simulink model "generic_wilmer_och_linnea_medvektorer2016b"  (R2016b)
settings: Solver=ode45  StartTime=0.0  StopTime=inf  RelTol=1e-3  EnableMultiTasking=on
libraries: CarMaker4SL x84, simulink x2
(part 1 of 2)
settings Model: ExtModeAutoUpdateStatusClock=off  Creator=fh  LastModifiedBy=Jeder
settings DataIOCC: LimitDataPoints=on  SaveFormat=Array  SignalLoggingSaveFormat=ModelDataLogs  SignalLoggingName=sigsOut
settings OptimizationCC: BooleanDataType=off  ExpressionDepthLimit=2147483647  InitFltsAndDblsToZero=on  LifeSpan=inf
settings DebuggingCC: SaveWithParameterizedLinksMsg=none  UnderspecifiedInitializationDetection=Classic  MergeDetectMultiDrivingBlocksExec=none  SignalResolutionControl=TryResolveAllWithWarning  MultiTaskDSMMsg=warning  MultiTaskCondExecSysMsg=none  FcnCallInpInsideContextMsg=warning  StateNameClashWarn=warning  SFUnexpectedBacktrackingDiag=warning  SFNoUnconditionalDefaultTransitionDiag=warning  SFExecutionAtInitializationDiag=none
settings HardwareCC: ProdBitPerPointer=32  ProdBitPerSizeT=32  ProdBitPerPtrDiffT=32  ProdLargestAtomicFloat=None  ProdIntDivRoundTo=Undefined  ProdEndianess=Unspecified  ProdWordSize=32  ProdHWDeviceType=32-bit Generic  TargetBitPerPointer=64  TargetBitPerSizeT=64  TargetBitPerPtrDiffT=64  TargetLongLongMode=on  TargetIntDivRoundTo=Zero  TargetEndianess=LittleEndian  TargetWordSize=64  TargetHWDeviceType=MATLAB Host  ProdEqTarget=off
settings ModelReferenceCC: PropagateSignalLabelsOutOfModel=off
settings CodeAppCC: MaxIdLength=63
settings GRTTargetCC: TargetFcnLib=ansi_tfl_tmw.mat  TargetLangStandard=C89/C90 (ANSI)  GeneratePreprocessorConditionals=Disable all  CombineOutputUpdateFcns=off  GRTInterface=on
settings ConfigComp: CovMetricSettings=dw  CovHtmlReporting=on  CovSaveCumulativeToWorkspaceVar=on  CovSaveSingleToWorkspaceVar=on  CovExternalEMLEnable=off

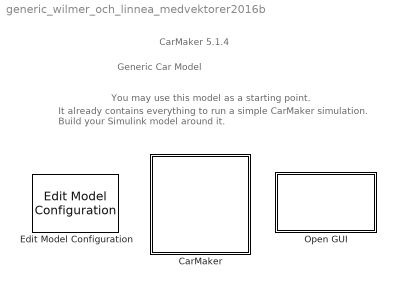
== system generic_wilmer_och_linnea_medvektorer2016b ==
  note: Generic Car Model
  note: You may use this model as a starting point.
  note: It already contains everything to run a simple CarMaker simulation.
      | Build your Simulink model around it.
  note: CarMaker 5.1.4
  CarMaker : Subsystem  TreatAsAtomicUnit=on
      mask Display: image(imread('CarMaker4SLss.bmp'));
  Edit Model Configuration : CarMaker4SL/Edit Model Configuration
  Open GUI : Subsystem  LoadFcn=if ~length(which('cmcmd')), cmenv; end
      settings: OpenFcn=cmblockmagic('gui_fix_display'); CM_Simulink
      mask Display: image(imread('CarMakerGUI.bmp'));

== system generic_wilmer_och_linnea_medvektorer2016b/CarMaker ==
  CM_FIRST : Subsystem
  CM_LAST : Subsystem
  DrivMan : Subsystem
  Ground : Ground
  IPG Vehicle : Subsystem  TreatAsAtomicUnit=on
  Terminator : Terminator
  VehicleControl : Subsystem
  wires:
  DrivMan/2(DrivMan.Out) -> VehicleControl/2(DrivMan.In)
  DrivMan/1(Sync_Out) -> VehicleControl/1(Sync_In)
  CM_FIRST/2(Env.Misc) -> DrivMan/2(Env.Misc)
  CM_FIRST/1(Sync_Out) -> DrivMan/1(Sync_In)
  CM_LAST/1(Sync_Out) -> Terminator/1
  IPG Vehicle/1(Sync_Out) -> CM_LAST/1(Sync_In)
  VehicleControl/1(Sync_Out) -> IPG Vehicle/1(Sync_In)
  VehicleControl/3(VhclCtrl.Steering) -> IPG Vehicle/3(VhclCtrl.Steering)
  VehicleControl/4(Vhcl.Wheel.In) -> IPG Vehicle/4(Vhcl.Wheel.In)
  VehicleControl/5(Vhcl.Misc) -> IPG Vehicle/5(Vhcl.Misc)
  VehicleControl/6(VhclCtrl.Brake) -> IPG Vehicle/6(VhclCtrl.Brake)
  VehicleControl/7(VhclCtrl.PT) -> IPG Vehicle/7(VhclCtrl.PT)
  VehicleControl/2(Vhcl.Model.Source) -> IPG Vehicle/2(Vhcl.Model.Source)
  Ground/1 -> CM_FIRST/1(Sync_In)

== system generic_wilmer_och_linnea_medvektorer2016b/Open GUI ==
  S-Function : S-Function  FunctionName=cm_gui  SFunctionDeploymentMode=off  EnableBusSupport=off

== system generic_wilmer_och_linnea_medvektorer2016b/CarMaker/CM_FIRST ==
  Sync_In : Inport
  Bus Creator1 : BusCreator  Inputs=9
  Demux : Demux  Outputs=9
  Environment : S-Function  FunctionName=CM_Sfun  Parameters='Environment'  SFunctionDeploymentMode=off  EnableBusSupport=off
  IoIn : S-Function  FunctionName=CM_Sfun  Parameters='IoIn'  SFunctionDeploymentMode=off  EnableBusSupport=off
  Sync_Out : Outport
  Env.Misc : Outport  Port=2
  wires:
  Bus Creator1/1 -> Env.Misc/1
  Environment/2 -> Demux/1
  Demux/4 -> Bus Creator1/4  "Env AirHumidity"
  Demux/3 -> Bus Creator1/3  "Env AirPressure"
  Demux/2 -> Bus Creator1/2  "Env AirDensity"
  Demux/1 -> Bus Creator1/1  "Env Temperature"
  Environment/1 -> Sync_Out/1
  IoIn/1 -> Environment/1
  Sync_In/1 -> IoIn/1
  Demux/5 -> Bus Creator1/5  "Env Time"
  Demux/6 -> Bus Creator1/6  "Env SolarRadiation"
  Demux/7 -> Bus Creator1/7  "Env WindVel_tot x"
  Demux/8 -> Bus Creator1/8  "Env WindVel_tot y"
  Demux/9 -> Bus Creator1/9  "Env WindVel_tot z"

== system generic_wilmer_och_linnea_medvektorer2016b/CarMaker/CM_LAST ==
  Sync_In : Inport
  CM_User : S-Function  FunctionName=CM_Sfun  Parameters='CM_User'  SFunctionDeploymentMode=off  EnableBusSupport=off
  IoOut : S-Function  FunctionName=CM_Sfun  Parameters='IoOut'  SFunctionDeploymentMode=off  EnableBusSupport=off
  Sync_Out : Outport
  wires:
  IoOut/1 -> Sync_Out/1
  CM_User/1 -> IoOut/1
  Sync_In/1 -> CM_User/1

== system generic_wilmer_och_linnea_medvektorer2016b/CarMaker/DrivMan ==
  note: There's rarely a reason to override DrivMan signals.
      | Use the VehicleControl interface for this purpose.
  Sync_In : Inport
  Env.Misc : Inport  Port=2
  BusCreator : BusCreator  Inputs=17
  Demux : Demux  Outputs=17
  DrivMan : S-Function  FunctionName=CM_Sfun  Parameters='DrivMan'  SFunctionDeploymentMode=off  EnableBusSupport=off
  Sync_Out : Outport
  DrivMan.Out : Outport  Port=2
  wires:
  Demux/17 -> BusCreator/17  "DrivMan Steering Trq"
  Demux/16 -> BusCreator/16  "DrivMan Steering AngAcc"
  Demux/15 -> BusCreator/15  "DrivMan Steering AngVel"
  Demux/14 -> BusCreator/14  "DrivMan Steering Ang"
  Demux/13 -> BusCreator/13  "DrivMan Gas"
  Demux/12 -> BusCreator/12  "DrivMan Clutch"
  Demux/11 -> BusCreator/11  "DrivMan BrakePark"
  Demux/10 -> BusCreator/10  "DrivMan Brake"
  Demux/9 -> BusCreator/9  "DrivMan GearNo"
  Demux/8 -> BusCreator/8  "DrivMan SelectorCtrl"
  Demux/7 -> BusCreator/7  "DrivMan UserSignal4"
  Demux/6 -> BusCreator/6  "DrivMan UserSignal3"
  Demux/5 -> BusCreator/5  "DrivMan UserSignal2"
  Demux/4 -> BusCreator/4  "DrivMan UserSignal1"
  Demux/3 -> BusCreator/3  "DrivMan UserSignal0"
  Demux/2 -> BusCreator/2  "DrivMan Key"
  Demux/1 -> BusCreator/1  "DrivMan SST"
  Env.Misc/1 -> DrivMan/2
  Sync_In/1 -> DrivMan/1
  DrivMan/1 -> Sync_Out/1
  BusCreator/1 -> DrivMan.Out/1
  DrivMan/2 -> Demux/1

== system generic_wilmer_och_linnea_medvektorer2016b/CarMaker/IPG Vehicle ==
  Sync_In : Inport
  Vhcl.Model.Source : Inport  Port=2
  VhclCtrl.Steering : Inport  Port=3
  Vhcl.Wheel.In : Inport  Port=4
  Vhcl.Misc : Inport  Port=5
  VhclCtrl.Brake : Inport  Port=6
  VhclCtrl.PT : Inport  Port=7
  Brake : Subsystem
  CarAndTrailer : Subsystem
  PowerTrain : Subsystem
  Stop Simulation : Stop
  VehicleSource_BuiltIn : simulink/Logic and Bit Operations/Compare To Constant  relop=~=  const=1  OutDataTypeStr=boolean  ZeroCross=off
  Sync_Out : Outport
  wires:
  VhclCtrl.PT/1 -> PowerTrain/3(VhclCtrl.PT)
  Brake/1(Sync_Out) -> PowerTrain/1(Sync_In)
  CarAndTrailer/1(Sync_Out) -> Brake/1(Sync_In)
  CarAndTrailer/2(Brake.IF.In) -> Brake/2(Brake.IF.In)
  VhclCtrl.Brake/1 -> Brake/3(VhclCtrl.Brake)
  PowerTrain/1(Sync_Out) -> Sync_Out/1
  Vhcl.Misc/1 -> CarAndTrailer/4(Vhcl.Misc)
  Vhcl.Wheel.In/1 -> CarAndTrailer/3(Vhcl.Wheel.In)
  VhclCtrl.Steering/1 -> CarAndTrailer/2(VhclCtrl.Steering)
  Sync_In/1 -> CarAndTrailer/1(Sync_In)
  Vhcl.Model.Source/1 -> VehicleSource_BuiltIn/1
  VehicleSource_BuiltIn/1 -> Stop Simulation/1
  Brake/2(Vhcl.Wheel.PT) -> PowerTrain/2(Vhcl.Wheel.PT)

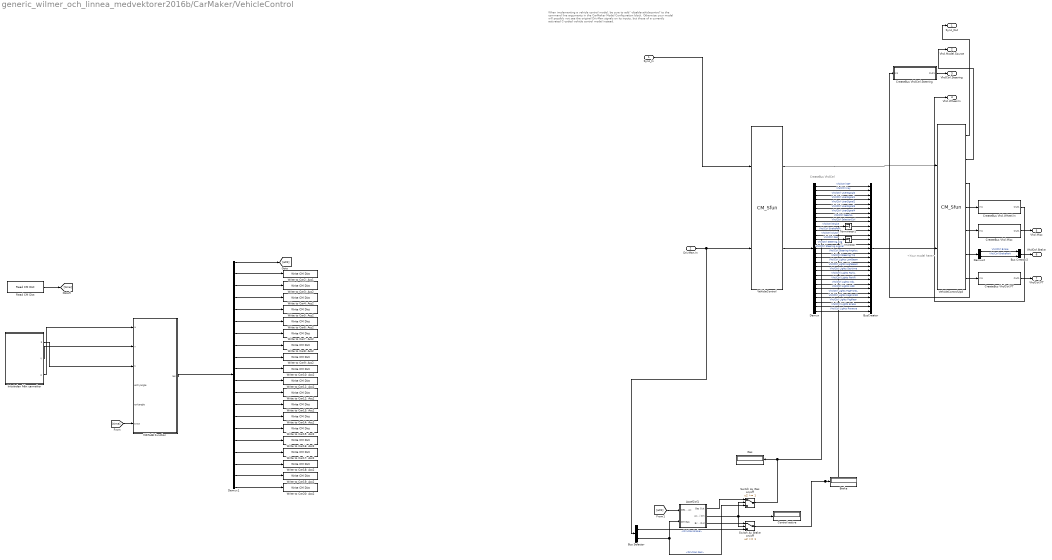
== system generic_wilmer_och_linnea_medvektorer2016b/CarMaker/VehicleControl ==
  note: CreateBus VhclCtrl
  note: <Your model here>
  note: When implementing a vehicle control model,
      | be sure to add '-disablevehiclecontrol' to the command line arguments
      | in the CarMaker Model Configuration block.
      | Otherwise your model will possibly not see the original DrivMan signals
      | on its inputs, but those of a currently activated C-coded vehicle control model instead.
  Sync_In : Inport
  DrivMan.In : Inport  Port=2
  AccelCtrl1 : Subsystem
  Brake : Display
  Bus Creator2 : BusCreator  Inputs=2
  Bus Selector : BusSelector  OutputSignals=DrivMan Brake,DrivMan Gas
  BusCreator : BusCreator  Inputs=29
  Control active : Display
  CreateBus Vhcl.Misc : Subsystem
  CreateBus Vhcl.Wheel.In : Subsystem
  CreateBus VhclCtrl.PT : Subsystem
  CreateBus VhclCtrl.Steering : Subsystem
  Demux : Demux  Outputs=29
  Demux1 : Demux  Outputs=20
  Demux2 : Demux  Outputs=2
  Gas : Display
  Initvärden från carmaker : Subsystem
  MATLAB Function : MATLAB Function  TreatAsAtomicUnit=on
  Read CM Dict : CarMaker4SL/Read CM Dict  xname=Time  xsync=off
  Switch Ax Brake on/off : Switch  Threshold=1  SaturateOnIntegerOverflow=on
  Switch Ax Gas on/off : Switch  Threshold=1  SaturateOnIntegerOverflow=on
  Terminator : Terminator
  Terminator1 : Terminator
  VehicleControl : S-Function  FunctionName=CM_Sfun  Parameters='VehicleControl'  SFunctionDeploymentMode=off  EnableBusSupport=off
  VehicleControlUpd : S-Function  FunctionName=CM_Sfun  Parameters='VehicleControlUpd'  SFunctionDeploymentMode=off  EnableBusSupport=off
  Write to Car10: Acc2 : CarMaker4SL/Write CM Dict  xname=Traffic.T08.LongAcc  xsync=off
  Write to Car11: Acc2 : CarMaker4SL/Write CM Dict  xname=Traffic.T09.LongAcc  xsync=off
  Write to Car12: Acc2 : CarMaker4SL/Write CM Dict  xname=Traffic.T10.LongAcc  xsync=off
  Write to Car13: Acc2 : CarMaker4SL/Write CM Dict  xname=Traffic.T11.LongAcc  xsync=off
  Write to Car14: Acc2 : CarMaker4SL/Write CM Dict  xname=Traffic.T12.LongAcc  xsync=off
  Write to Car15: Acc2 : CarMaker4SL/Write CM Dict  xname=Traffic.T13.LongAcc  xsync=off
  Write to Car16: Acc2 : CarMaker4SL/Write CM Dict  xname=Traffic.T14.LongAcc  xsync=off
  Write to Car17: Acc2 : CarMaker4SL/Write CM Dict  xname=Traffic.T15.LongAcc  xsync=off
  Write to Car18: Acc2 : CarMaker4SL/Write CM Dict  xname=Traffic.T16.LongAcc  xsync=off
  Write to Car19: Acc2 : CarMaker4SL/Write CM Dict  xname=Traffic.T17.LongAcc  xsync=off
  Write to Car20: Acc2 : CarMaker4SL/Write CM Dict  xname=Traffic.T18.LongAcc  xsync=off
  Write to Car2: Acc1 : CarMaker4SL/Write CM Dict  xname=Traffic.T00.LongAcc  xsync=off
  Write to Car3: Acc2 : CarMaker4SL/Write CM Dict  xname=Traffic.T01.LongAcc  xsync=off
  Write to Car4: Acc2 : CarMaker4SL/Write CM Dict  xname=Traffic.T02.LongAcc  xsync=off
  Write to Car5: Acc2 : CarMaker4SL/Write CM Dict  xname=Traffic.T03.LongAcc  xsync=off
  Write to Car6: Acc2 : CarMaker4SL/Write CM Dict  xname=Traffic.T04.LongAcc  xsync=off
  Write to Car7: Acc2 : CarMaker4SL/Write CM Dict  xname=Traffic.T05.LongAcc  xsync=off
  Write to Car8: Acc2 : CarMaker4SL/Write CM Dict  xname=Traffic.T06.LongAcc  xsync=off
  Write to Car9: Acc2 : CarMaker4SL/Write CM Dict  xname=Traffic.T07.LongAcc  xsync=off
  Sync_Out : Outport
  Vhcl.Model.Source : Outport  Port=2
  VhclCtrl.Steering : Outport  Port=3
  Vhcl.Wheel.In : Outport  Port=4
  Vhcl.Misc : Outport  Port=5
  VhclCtrl.Brake : Outport  Port=6
  VhclCtrl.PT : Outport  Port=7
  wires:
  BusCreator/1 -> VehicleControlUpd/2
  VehicleControlUpd/2 -> Vhcl.Model.Source/1
  VehicleControlUpd/4 -> CreateBus Vhcl.Wheel.In/1(In1)
  VehicleControlUpd/5 -> CreateBus Vhcl.Misc/1(In1)
  VehicleControlUpd/6 -> Demux2/1
  VehicleControlUpd/7 -> CreateBus VhclCtrl.PT/1(In1)
  VehicleControlUpd/3 -> CreateBus VhclCtrl.Steering/1(In1)
  CreateBus Vhcl.Misc/1(Out1) -> Vhcl.Misc/1
  CreateBus Vhcl.Wheel.In/1(Out1) -> Vhcl.Wheel.In/1
  VehicleControl/1 -> VehicleControlUpd/1
  Sync_In/1 -> VehicleControl/1
  CreateBus VhclCtrl.PT/1(Out1) -> VhclCtrl.PT/1
  Bus Creator2/1 -> VhclCtrl.Brake/1
  CreateBus VhclCtrl.Steering/1(Out1) -> VhclCtrl.Steering/1
  VehicleControlUpd/1 -> Sync_Out/1
  Demux2/2 -> Bus Creator2/2  "VhclCtrl BrakePark"
  Demux2/1 -> Bus Creator2/1  "VhclCtrl Brake"
  Demux/29 -> BusCreator/29  "VhclCtrl Lights Reverse"
  Demux/28 -> BusCreator/28  "VhclCtrl Lights Brake"
  Demux/27 -> BusCreator/27  "VhclCtrl Lights FogRear"
  Demux/26 -> BusCreator/26  "VhclCtrl Lights FogFrontR"
  Demux/25 -> BusCreator/25  "VhclCtrl Lights FogFrontL"
  Demux/24 -> BusCreator/24  "VhclCtrl Lights IndR"
  Demux/23 -> BusCreator/23  "VhclCtrl Lights IndL"
  Demux/22 -> BusCreator/22  "VhclCtrl Lights ParkR"
  Demux/21 -> BusCreator/21  "VhclCtrl Lights ParkL"
  Demux/20 -> BusCreator/20  "VhclCtrl Lights Daytime"
  Demux/19 -> BusCreator/19  "VhclCtrl Lights HighBeam"
  Demux/18 -> BusCreator/18  "VhclCtrl Lights LowBeam"
  Demux/17 -> BusCreator/17  "VhclCtrl Steering Trq"
  Demux/16 -> BusCreator/16  "VhclCtrl Steering AngAcc"
  Demux/15 -> BusCreator/15  "VhclCtrl Steering AngVel"
  Demux/14 -> BusCreator/14  "VhclCtrl Steering Ang"
  Demux/13 -> Terminator/1  "VhclCtrl Gas"
  Demux/12 -> BusCreator/12  "VhclCtrl Clutch"
  Demux/11 -> BusCreator/11  "VhclCtrl BrakePark"
  Demux/10 -> Terminator1/1  "VhclCtrl Brake"
  Demux/9 -> BusCreator/9  "VhclCtrl SelectorCtrl"
  Demux/8 -> BusCreator/8  "VhclCtrl GearNo"
  Demux/7 -> BusCreator/7  "VhclCtrl UserSignal4"
  Demux/6 -> BusCreator/6  "VhclCtrl UserSignal3"
  Demux/5 -> BusCreator/5  "VhclCtrl UserSignal2"
  Demux/4 -> BusCreator/4  "VhclCtrl UserSignal1"
  Demux/3 -> BusCreator/3  "VhclCtrl UserSignal0"
  Demux/2 -> BusCreator/2  "VhclCtrl Key"
  Demux/1 -> BusCreator/1  "VhclCtrl SST"
  VehicleControl/2 -> Demux/1
  DrivMan.In/1 -> VehicleControl/2, Bus Selector/1
  AccelCtrl1/2(AxCtrl On) -> Switch Ax Gas on/off/2, Control active/1, Switch Ax Brake on/off/2
  Bus Selector/1 -> Switch Ax Brake on/off/3  "<DrivMan Brake>"
  AccelCtrl1/3(Brake Out) -> Switch Ax Brake on/off/1
  AccelCtrl1/1(Gas Out) -> Switch Ax Gas on/off/1
  Bus Selector/2 -> Switch Ax Gas on/off/3, AccelCtrl1/2(DM Gas)  "<DrivMan Gas>"
  [a01] -> AccelCtrl1/1(Desired Ax)
  Switch Ax Gas on/off/1 -> BusCreator/13, Gas/1
  Switch Ax Brake on/off/1 -> Brake/1, BusCreator/10
  MATLAB Function/1(res) -> Demux1/1
  Initvärden från carmaker/1("S ") -> MATLAB Function/3(s)
  Initvärden från carmaker/2("V ") -> MATLAB Function/2(v)
  Initvärden från carmaker/3("A ") -> MATLAB Function/1(a)
  Demux1/1 -> [a01]
  Demux1/2 -> Write to Car2: Acc1/1
  Demux1/3 -> Write to Car3: Acc2/1
  Demux1/4 -> Write to Car4: Acc2/1
  Demux1/5 -> Write to Car5: Acc2/1
  Demux1/6 -> Write to Car6: Acc2/1
  Demux1/7 -> Write to Car7: Acc2/1
  Demux1/8 -> Write to Car8: Acc2/1
  Demux1/9 -> Write to Car9: Acc2/1
  Demux1/10 -> Write to Car10: Acc2/1
  Demux1/11 -> Write to Car11: Acc2/1
  Demux1/12 -> Write to Car12: Acc2/1
  Demux1/13 -> Write to Car13: Acc2/1
  Demux1/14 -> Write to Car14: Acc2/1
  Demux1/15 -> Write to Car15: Acc2/1
  Demux1/16 -> Write to Car16: Acc2/1
  Demux1/17 -> Write to Car17: Acc2/1
  Demux1/18 -> Write to Car18: Acc2/1
  Demux1/19 -> Write to Car19: Acc2/1
  Demux1/20 -> Write to Car20: Acc2/1
  Read CM Dict/1 -> [time]
  [time] -> MATLAB Function/6(time)

== system generic_wilmer_och_linnea_medvektorer2016b/CarMaker/IPG Vehicle/Brake ==
  note: <Your model here>
  note: When replacing the entire braking system,
      | be sure to add '-disablebrake' to the command line arguments
      | in the CarMaker Model Configuration block.
  Sync_In : Inport
  Brake.IF.In : Inport  Port=2
  VhclCtrl.Brake : Inport  Port=3
  Brake : S-Function  FunctionName=CM_Sfun  Parameters='Brake'  SFunctionDeploymentMode=off  EnableBusSupport=off
  BrakeUpd : S-Function  FunctionName=CM_Sfun  Parameters='BrakeUpd'  SFunctionDeploymentMode=off  EnableBusSupport=off
  BusCreator : BusCreator  Inputs=12
  CreateBus Vhcl.Wheel.PT : Subsystem
  Demux : Demux  Outputs=12
  Sync_Out : Outport
  Vhcl.Wheel.PT : Outport  Port=2
  wires:
  BrakeUpd/1 -> Sync_Out/1
  Brake/1 -> BrakeUpd/1  "Sync"
  Brake.IF.In/1 -> Brake/2
  VhclCtrl.Brake/1 -> Brake/3
  Brake/2 -> Demux/1
  BusCreator/1 -> BrakeUpd/2
  Sync_In/1 -> Brake/1
  Demux/12 -> BusCreator/12  "Brake IF Trq_Reg_trg RR"
  Demux/11 -> BusCreator/11  "Brake IF Trq_Reg_trg RL"
  Demux/10 -> BusCreator/10  "Brake IF Trq_Reg_trg FR"
  Demux/9 -> BusCreator/9  "Brake IF Trq_Reg_trg FL"
  Demux/8 -> BusCreator/8  "Brake IF Trq_PB RR"
  Demux/7 -> BusCreator/7  "Brake IF Trq_PB RL"
  Demux/6 -> BusCreator/6  "Brake IF Trq_PB FR"
  Demux/5 -> BusCreator/5  "Brake IF Trq_PB FL"
  Demux/4 -> BusCreator/4  "Brake IF Trq_WB RR"
  Demux/3 -> BusCreator/3  "Brake IF Trq_WB RL"
  Demux/2 -> BusCreator/2  "Brake IF Trq_WB FR"
  Demux/1 -> BusCreator/1  "Brake IF Trq_WB FL"
  BrakeUpd/2 -> CreateBus Vhcl.Wheel.PT/1(In)
  CreateBus Vhcl.Wheel.PT/1(Out) -> Vhcl.Wheel.PT/1

== system generic_wilmer_och_linnea_medvektorer2016b/CarMaker/IPG Vehicle/CarAndTrailer ==
  Sync_In : Inport
  VhclCtrl.Steering : Inport  Port=2
  Vhcl.Wheel.In : Inport  Port=3
  Vhcl.Misc : Inport  Port=4
  CarAndTrailerUpd : Subsystem
  Forces : Subsystem
  Ground : Ground
  Kinematics : Subsystem
  Kinetics : Subsystem
  Steering : Subsystem
  Terminator : Terminator
  Terminator1 : Terminator
  Trailer : Subsystem
  Sync_Out : Outport
  Brake.IF.In : Outport  Port=2
  wires:
  Trailer/9(Car.Hitch.FrcTrq) -> CarAndTrailerUpd/9(Car.Hitch.FrcTrq)
  Trailer/8(Vhcl.Wheel.RR) -> CarAndTrailerUpd/8(Vhcl.Wheel.RR)
  Trailer/7(Vhcl.Wheel.RL) -> CarAndTrailerUpd/7(Vhcl.Wheel.RL)
  Trailer/6(Vhcl.Wheel.FR) -> CarAndTrailerUpd/6(Vhcl.Wheel.FR)
  Trailer/5(Vhcl.Wheel.FL) -> CarAndTrailerUpd/5(Vhcl.Wheel.FL)
  Trailer/4(Vhcl.PoI) -> CarAndTrailerUpd/4(Vhcl.PoI)
  Trailer/3(Vhcl.Motion) -> CarAndTrailerUpd/3(Vhcl.Motion)
  Trailer/2(Vhcl.Steering) -> CarAndTrailerUpd/2(Vhcl.Steering)
  Trailer/1(Sync_Out) -> CarAndTrailerUpd/1(Sync_In)
  CarAndTrailerUpd/2(Brake.IF.In) -> Brake.IF.In/1
  CarAndTrailerUpd/1(Sync_Out) -> Sync_Out/1
  Vhcl.Misc/1 -> Terminator1/1
  Vhcl.Wheel.In/1 -> Terminator/1
  Kinetics/6(WheelCarrier.Misc) -> Trailer/6(WheelCarrier.Misc)
  Kinetics/5(Car.Trq_T2W) -> Trailer/5(Car.Trq_T2W)
  Steering/2(Steer.IF) -> Kinematics/2(Steer.IF)
  Kinetics/4(Car.Fr1) -> Trailer/4(Car.Fr1)
  Kinetics/3(Car.Hitch) -> Trailer/3(Car.Hitch)
  Kinetics/2(Trailer.Load) -> Trailer/2(Trailer.Load)
  VhclCtrl.Steering/1 -> Steering/2(VhclCtrl.Steering)
  Sync_In/1 -> Steering/1(Sync_In)
  Steering/1(Sync_Out) -> Kinematics/1(Sync_In)
  Kinetics/1(Sync_Out) -> Trailer/1(Sync_In)
  Ground/1 -> CarAndTrailerUpd/10(Vhcl.Fr1A)
  Forces/11(FStabi) -> Kinetics/11(FStabi)
  Forces/10(FDamp) -> Kinetics/10(FDamp)
  Forces/9(FSpring) -> Kinetics/9(FSpring)
  Forces/8(TireRR_Out) -> Kinetics/8(TireRR.Out)
  Forces/7(TireRL_Out) -> Kinetics/7(TireRL.Out)
  Forces/6(TireFR_Out) -> Kinetics/6(TireFR.Out)
  Forces/5(TireFL_Out) -> Kinetics/5(TireFL.Out)
  Forces/4(Car.Load) -> Kinetics/4(Car.Load)
  Forces/2(Car.Virtual) -> Kinetics/2(Car.Virtual)
  Kinematics/6(lSpring) -> Forces/6(lSpring)
  Kinematics/7(vDamp) -> Forces/7(vDamp)
  Forces/3(Car.Aero) -> Kinetics/3(Car.Aero)
  Forces/1(Sync_Out) -> Kinetics/1(Sync_In)
  Kinematics/5(TireRR_In) -> Forces/5(TireRR_In)
  Kinematics/4(TireRL_In) -> Forces/4(TireRL_In)
  Kinematics/3(TireFR_In) -> Forces/3(TireFR_In)
  Kinematics/2(TireFL_In) -> Forces/2(TireFL_In)
  Kinematics/1(Sync_Out) -> Forces/1(Sync_In)
  Kinematics/8(lStabi) -> Forces/8(lStabi)
  Forces/12(FBuf) -> Kinetics/12(FBuf)
  Kinematics/9(lBuf) -> Forces/9(lBuf)

== system generic_wilmer_och_linnea_medvektorer2016b/CarMaker/IPG Vehicle/PowerTrain ==
  note: When replacing the entire powertrain,
      | be sure to add '-disablepowertrain' to the command line arguments
      | in the CarMaker Model Configuration block.
  note: <Your model here>
  Sync_In : Inport
  Vhcl.Wheel.PT : Inport  Port=2
  VhclCtrl.PT : Inport  Port=3
  BusCreator : BusCreator  Inputs=40
  Demux : Demux  Outputs=40
  PowerTrain : S-Function  FunctionName=CM_Sfun  Parameters='PowerTrain'  SFunctionDeploymentMode=off  EnableBusSupport=off
  PowerTrainUpd : S-Function  FunctionName=CM_Sfun  Parameters='PowerTrainUpd'  SFunctionDeploymentMode=off  EnableBusSupport=off
  Sync_Out : Outport
  wires:
  Sync_In/1 -> PowerTrain/1
  PowerTrain/2 -> Demux/1
  PowerTrainUpd/1 -> Sync_Out/1
  PowerTrain/1 -> PowerTrainUpd/1  "Sync"
  BusCreator/1 -> PowerTrainUpd/2
  Demux/1 -> BusCreator/1  "PT IF Ignition"
  Demux/2 -> BusCreator/2  "PT IF OperationState"
  Demux/3 -> BusCreator/3  "PT IF OperationError"
  Demux/4 -> BusCreator/4  "PT IF GearNo"
  Demux/5 -> BusCreator/5  "PT IF Engine_rotv"
  Demux/6 -> BusCreator/6  "PT IF Engine_Trq (EngineControl)"
  Demux/7 -> BusCreator/7  "PT IF Trq_Supp2Bdy1 x"
  Demux/8 -> BusCreator/8  "PT IF Trq_Supp2Bdy1 y"
  Demux/9 -> BusCreator/9  "PT IF Trq_Supp2Bdy1 z"
  Demux/10 -> BusCreator/10  "PT IF Trq_Supp2BdyEng x"
  Demux/11 -> BusCreator/11  "PT IF Trq_Supp2BdyEng y"
  Demux/12 -> BusCreator/12  "PT IF DL_iDiff_mean"
  Demux/13 -> BusCreator/13  "PT IF WFL rot"
  Demux/14 -> BusCreator/14  "PT IF WFL rotv"
  Demux/15 -> BusCreator/15  "PT IF WFL Trq_B2W"
  Demux/16 -> BusCreator/16  "PT IF WFL Trq_Drive"
  Demux/17 -> BusCreator/17  "PT IF WFL Trq_Supp2WC"
  Demux/18 -> BusCreator/18  "PT IF WFL Trq_BrakeReg"
  Demux/19 -> BusCreator/19  "PT IF WFL Trq_BrakeReg_max"
  Demux/20 -> BusCreator/20  "PT IF WFR rot"
  Demux/21 -> BusCreator/21  "PT IF WFR rotv"
  Demux/22 -> BusCreator/22  "PT IF WFR Trq_B2W"
  Demux/23 -> BusCreator/23  "PT IF WFR Trq_Drive"
  Demux/24 -> BusCreator/24  "PT IF WFR Trq_Supp2WC"
  Demux/25 -> BusCreator/25  "PT IF WFR Trq_BrakeReg"
  Demux/26 -> BusCreator/26  "PT IF WFR Trq_BrakeReg_max"
  Demux/27 -> BusCreator/27  "PT IF WRL rot"
  Demux/28 -> BusCreator/28  "PT IF WRL rotv"
  Demux/29 -> BusCreator/29  "PT IF WRL Trq_B2W"
  Demux/30 -> BusCreator/30  "PT IF WRL Trq_Drive"
  Demux/31 -> BusCreator/31  "PT IF WRL Trq_Supp2WC"
  Demux/32 -> BusCreator/32  "PT IF WRL Trq_BrakeReg"
  Demux/33 -> BusCreator/33  "PT IF WRL Trq_BrakeReg_max"
  Demux/34 -> BusCreator/34  "PT IF WRR rot"
  Demux/35 -> BusCreator/35  "PT IF WRR rotv"
  Demux/36 -> BusCreator/36  "PT IF WRR Trq_B2W"
  Demux/37 -> BusCreator/37  "PT IF WRR Trq_Drive"
  Demux/38 -> BusCreator/38  "PT IF WRR Trq_Supp2WC"
  Demux/39 -> BusCreator/39  "PT IF WRR Trq_BrakeReg"
  Demux/40 -> BusCreator/40  "PT IF WRR Trq_BrakeReg_max"
  VhclCtrl.PT/1 -> PowerTrain/3
  Vhcl.Wheel.PT/1 -> PowerTrain/2

== system generic_wilmer_och_linnea_medvektorer2016b/CarMaker/VehicleControl/AccelCtrl1 ==
  note: x
  note: x
  Desired Ax : Inport
  DM Gas : Inport  Port=2
  Brake if -1<x<0 : Saturate  UpperLimit=0  LowerLimit=-1
  Compare To Constant : simulink/Logic and Bit Operations/Compare To Constant  relop=~=  const=0  OutDataTypeStr=boolean
  Gain : Gain  Gain=-1  SaturateOnIntegerOverflow=on  OutDataTypeStr=Inherit: Same as input  ParamDataTypeStr=Inherit: Same as input
  Gas  if 0<=x<=1 : Saturate  UpperLimit=1  LowerLimit=0
  PI-Controller : Subsystem
  "controlled process variable " : Subsystem
  Gas Out : Outport
  AxCtrl On : Outport  Port=2
  Brake Out : Outport  Port=3
  wires:
  Compare To Constant/1 -> AxCtrl On/1, PI-Controller/3(AxCtrl On)
  Brake if -1<x<0/1 -> Gain/1
  Gas  if 0<=x<=1/1 -> Gas Out/1
  PI-Controller/1(Gas or Brake) -> Gas  if 0<=x<=1/1, Brake if -1<x<0/1
  DM Gas/1 -> PI-Controller/2(DM_Gas)
  "controlled process variable "/1(delta ax) -> PI-Controller/1(delta_ax)
  Gain/1 -> Brake Out/1
  Desired Ax/1 -> "controlled process variable "/1(desired ax), Compare To Constant/1

== system generic_wilmer_och_linnea_medvektorer2016b/CarMaker/VehicleControl/CreateBus Vhcl.Misc ==
  In1 : Inport
  Bus Creator5 : BusCreator  Inputs=11
  Demux5 : Demux  Outputs=11
  Out1 : Outport
  wires:
  Demux5/11 -> Bus Creator5/11  "Vhcl Wind_vel_0 z"
  Demux5/10 -> Bus Creator5/10  "Vhcl Wind_vel_0 y"
  Demux5/9 -> Bus Creator5/9  "Vhcl Wind_vel_0 x"
  Demux5/8 -> Bus Creator5/8  "Vhcl DL2BdyEng y"
  Demux5/7 -> Bus Creator5/7  "Vhcl DL2BdyEng x"
  Demux5/6 -> Bus Creator5/6  "Vhcl TrqDL2Bdy1B z"
  Demux5/5 -> Bus Creator5/5  "Vhcl TrqDL2Bdy1B y"
  Demux5/4 -> Bus Creator5/4  "Vhcl TrqDL2Bdy1B x"
  Demux5/3 -> Bus Creator5/3  "Vhcl Trq_DL2Bdy1 z"
  In1/1 -> Demux5/1
  Bus Creator5/1 -> Out1/1
  Demux5/2 -> Bus Creator5/2  "Vhcl Trq_DL2Bdy1 y"
  Demux5/1 -> Bus Creator5/1  "Vhcl Trq_DL2Bdy1 x"

== system generic_wilmer_och_linnea_medvektorer2016b/CarMaker/VehicleControl/CreateBus Vhcl.Wheel.In ==
  In1 : Inport
  Bus Creator1 : BusCreator  Inputs=12
  Demux1 : Demux  Outputs=12
  Out1 : Outport
  wires:
  Demux1/12 -> Bus Creator1/12  "Vhcl Wheel RR rotv"
  Demux1/11 -> Bus Creator1/11  "Vhcl Wheel RR Trq_DL2WC"
  Demux1/10 -> Bus Creator1/10  "Vhcl Wheel RR Trq_B2WC"
  Demux1/9 -> Bus Creator1/9  "Vhcl Wheel RL rotv"
  Demux1/8 -> Bus Creator1/8  "Vhcl Wheel RL Trq_DL2WC"
  Demux1/7 -> Bus Creator1/7  "Vhcl Wheel RL Trq_B2WC"
  Demux1/6 -> Bus Creator1/6  "Vhcl Wheel FR rotv"
  Demux1/5 -> Bus Creator1/5  "Vhcl Wheel FR Trq_DL2WC"
  Demux1/4 -> Bus Creator1/4  "Vhcl Wheel FR Trq_B2WC"
  Demux1/3 -> Bus Creator1/3  "Vhcl Wheel FL rotv"
  In1/1 -> Demux1/1
  Bus Creator1/1 -> Out1/1
  Demux1/2 -> Bus Creator1/2  "Vhcl Wheel FL Trq_DL2WC"
  Demux1/1 -> Bus Creator1/1  "Vhcl Wheel FL Trq_B2WC"

== system generic_wilmer_och_linnea_medvektorer2016b/CarMaker/VehicleControl/CreateBus VhclCtrl.PT ==
  In1 : Inport
  BusCreator : BusCreator  Inputs=11
  Demux : Demux  Outputs=11
  Out1 : Outport
  wires:
  In1/1 -> Demux/1
  BusCreator/1 -> Out1/1
  Demux/1 -> BusCreator/1  "VhclCtrl SST"
  Demux/2 -> BusCreator/2  "VhclCtrl Key"
  Demux/3 -> BusCreator/3  "VhclCtrl UserSignal0"
  Demux/4 -> BusCreator/4  "VhclCtrl UserSignal1"
  Demux/5 -> BusCreator/5  "VhclCtrl UserSignal2"
  Demux/6 -> BusCreator/6  "VhclCtrl UserSignal3"
  Demux/7 -> BusCreator/7  "VhclCtrl UserSignal4"
  Demux/8 -> BusCreator/8  "VhclCtrl GearNo"
  Demux/9 -> BusCreator/9  "VhclCtrl SelectorCtrl"
  Demux/10 -> BusCreator/10  "VhclCtrl Clutch"
  Demux/11 -> BusCreator/11  "VhclCtrl Gas"

== system generic_wilmer_och_linnea_medvektorer2016b/CarMaker/VehicleControl/CreateBus VhclCtrl.Steering ==
  In1 : Inport
  Bus Creator : BusCreator  Inputs=5
  Demux : Demux  Outputs=5
  Out1 : Outport
  wires:
  In1/1 -> Demux/1
  Bus Creator/1 -> Out1/1
  Demux/1 -> Bus Creator/1  "VhclCtrl Steering Ang"
  Demux/5 -> Bus Creator/5  "VhclCtrl Steering ByTrq"
  Demux/3 -> Bus Creator/3  "VhclCtrl Steering AngAcc"
  Demux/2 -> Bus Creator/2  "VhclCtrl Steering AngVel"
  Demux/4 -> Bus Creator/4  "VhclCtrl Steering Trq"

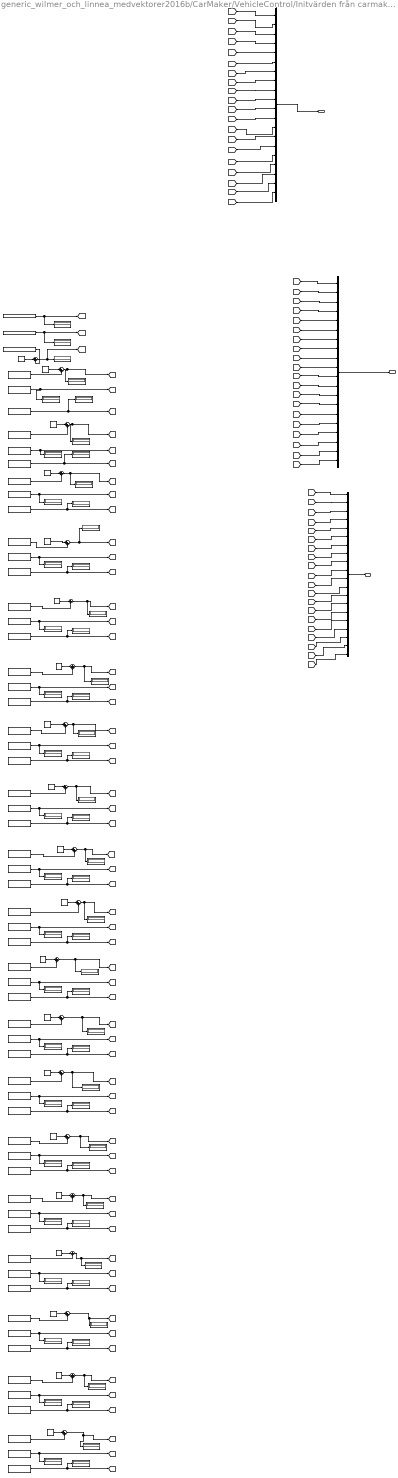
== system generic_wilmer_och_linnea_medvektorer2016b/CarMaker/VehicleControl/Initvärden från carmaker ==
  Constant{,1..19} (20 alike) : Constant  Value=-145
  Display{,1..56} (57 alike) : Display
  Mux : Mux  Inputs=20
  Mux1 : Mux  Inputs=20
  Mux2 : Mux  Inputs=20
  Read CM acceleration : CarMaker4SL/Read CM Dict  xname=Car.ax  xsync=off
  "Read CM position " : CarMaker4SL/Read CM Dict  xname=Car.Road.sRoad  xsync=off
  Read CM velocity : CarMaker4SL/Read CM Dict  xname=Car.vx  xsync=off
  Read Car10 acc : CarMaker4SL/Read CM Dict  xname=Traffic.T08.LongAcc  xsync=off
  Read Car10 dist : CarMaker4SL/Read CM Dict  xname=Traffic.T08.sRoad  xsync=off
  Read Car10 vel : CarMaker4SL/Read CM Dict  xname=Traffic.T08.LongVel  xsync=off
  Read Car11 acc : CarMaker4SL/Read CM Dict  xname=Traffic.T09.LongAcc  xsync=off
  Read Car11 dist : CarMaker4SL/Read CM Dict  xname=Traffic.T09.sRoad  xsync=off
  Read Car11 vel : CarMaker4SL/Read CM Dict  xname=Traffic.T09.LongVel  xsync=off
  Read Car12 acc : CarMaker4SL/Read CM Dict  xname=Traffic.T10.LongAcc  xsync=off
  Read Car12 dist : CarMaker4SL/Read CM Dict  xname=Traffic.T10.sRoad  xsync=off
  Read Car12 vel : CarMaker4SL/Read CM Dict  xname=Traffic.T10.LongVel  xsync=off
  Read Car13 acc : CarMaker4SL/Read CM Dict  xname=Traffic.T11.LongAcc  xsync=off
  Read Car13 dist : CarMaker4SL/Read CM Dict  xname=Traffic.T11.sRoad  xsync=off
  Read Car13 vel : CarMaker4SL/Read CM Dict  xname=Traffic.T11.LongVel  xsync=off
  Read Car14 acc : CarMaker4SL/Read CM Dict  xname=Traffic.T12.LongAcc  xsync=off
  Read Car14 dist : CarMaker4SL/Read CM Dict  xname=Traffic.T12.sRoad  xsync=off
  Read Car14 vel : CarMaker4SL/Read CM Dict  xname=Traffic.T12.LongVel  xsync=off
  Read Car15 acc : CarMaker4SL/Read CM Dict  xname=Traffic.T13.LongAcc  xsync=off
  Read Car15 dist : CarMaker4SL/Read CM Dict  xname=Traffic.T13.sRoad  xsync=off
  Read Car15 vel : CarMaker4SL/Read CM Dict  xname=Traffic.T13.LongVel  xsync=off
  Read Car16 acc : CarMaker4SL/Read CM Dict  xname=Traffic.T14.LongAcc  xsync=off
  Read Car16 dist : CarMaker4SL/Read CM Dict  xname=Traffic.T14.sRoad  xsync=off
  Read Car16 vel : CarMaker4SL/Read CM Dict  xname=Traffic.T14.LongVel  xsync=off
  Read Car17 acc : CarMaker4SL/Read CM Dict  xname=Traffic.T15.LongAcc  xsync=off
  Read Car17 dist : CarMaker4SL/Read CM Dict  xname=Traffic.T15.sRoad  xsync=off
  Read Car17 vel : CarMaker4SL/Read CM Dict  xname=Traffic.T15.LongVel  xsync=off
  Read Car18 acc : CarMaker4SL/Read CM Dict  xname=Traffic.T16.LongAcc  xsync=off
  Read Car18 dist : CarMaker4SL/Read CM Dict  xname=Traffic.T16.sRoad  xsync=off
  Read Car18 vel : CarMaker4SL/Read CM Dict  xname=Traffic.T16.LongVel  xsync=off
  Read Car19 acc : CarMaker4SL/Read CM Dict  xname=Traffic.T17.LongAcc  xsync=off
  Read Car19 dist : CarMaker4SL/Read CM Dict  xname=Traffic.T17.sRoad  xsync=off
  Read Car19 vel : CarMaker4SL/Read CM Dict  xname=Traffic.T17.LongVel  xsync=off
  Read Car2 acc : CarMaker4SL/Read CM Dict  xname=Traffic.T00.LongAcc  xsync=off
  Read Car2 dist : CarMaker4SL/Read CM Dict  xname=Traffic.T00.sRoad  xsync=off
  Read Car2 m/s : CarMaker4SL/Read CM Dict  xname=Traffic.T00.LongVel  xsync=off
  Read Car20 acc : CarMaker4SL/Read CM Dict  xname=Traffic.T18.LongAcc  xsync=off
  Read Car20 dist : CarMaker4SL/Read CM Dict  xname=Traffic.T18.sRoad  xsync=off
  Read Car20 vel : CarMaker4SL/Read CM Dict  xname=Traffic.T18.LongVel  xsync=off
  Read Car3 acc : CarMaker4SL/Read CM Dict  xname=Traffic.T01.LongAcc  xsync=off
  Read Car3 dist : CarMaker4SL/Read CM Dict  xname=Traffic.T01.sRoad  xsync=off
  Read Car3 vel : CarMaker4SL/Read CM Dict  xname=Traffic.T01.LongVel  xsync=off
  Read Car4 acc : CarMaker4SL/Read CM Dict  xname=Traffic.T02.LongAcc  xsync=off
  Read Car4 dist : CarMaker4SL/Read CM Dict  xname=Traffic.T02.sRoad  xsync=off
  Read Car4 vel : CarMaker4SL/Read CM Dict  xname=Traffic.T02.LongVel  xsync=off
  Read Car5 acc5 : CarMaker4SL/Read CM Dict  xname=Traffic.T03.LongAcc  xsync=off
  Read Car5 dist : CarMaker4SL/Read CM Dict  xname=Traffic.T03.sRoad  xsync=off
  Read Car5 vel5 : CarMaker4SL/Read CM Dict  xname=Traffic.T03.LongVel  xsync=off
  Read Car6 acc : CarMaker4SL/Read CM Dict  xname=Traffic.T04.LongAcc  xsync=off
  Read Car6 dist : CarMaker4SL/Read CM Dict  xname=Traffic.T04.sRoad  xsync=off
  Read Car6 vel : CarMaker4SL/Read CM Dict  xname=Traffic.T04.LongVel  xsync=off
  Read Car7 acc1 : CarMaker4SL/Read CM Dict  xname=Traffic.T05.LongAcc  xsync=off
  Read Car7 dist1 : CarMaker4SL/Read CM Dict  xname=Traffic.T05.sRoad  xsync=off
  Read Car7 vel1 : CarMaker4SL/Read CM Dict  xname=Traffic.T05.LongVel  xsync=off
  Read Car8 acc : CarMaker4SL/Read CM Dict  xname=Traffic.T06.LongAcc  xsync=off
  Read Car8 dist : CarMaker4SL/Read CM Dict  xname=Traffic.T06.sRoad  xsync=off
  Read Car8 vel : CarMaker4SL/Read CM Dict  xname=Traffic.T06.LongVel  xsync=off
  Read Car9 acc : CarMaker4SL/Read CM Dict  xname=Traffic.T07.LongAcc  xsync=off
  Read Car9 dist : CarMaker4SL/Read CM Dict  xname=Traffic.T07.sRoad  xsync=off
  Read Car9 vel : CarMaker4SL/Read CM Dict  xname=Traffic.T07.LongVel  xsync=off
  Sum{,1..19} (20 alike) : Sum  Inputs=|++
  pos : Display
  vx1 : Display
  vx2 : Display
  "S " : Outport
  "V " : Outport  Port=2
  "A " : Outport  Port=3
  wires:
  Read Car2 acc/1 -> [a2], Display/1
  Read Car4 vel/1 -> [v4], Display6/1
  Read Car4 acc/1 -> [a4], Display7/1
  Read Car3 acc/1 -> [a3], Display5/1
  Read Car3 vel/1 -> Display4/1, [v3]
  Read Car2 m/s/1 -> Display2/1, [v2]
  Read Car2 dist/1 -> Sum1/2
  Read Car3 dist/1 -> Sum2/2
  Read Car4 dist/1 -> Sum3/2
  Read Car5 vel5/1 -> [v5], Display9/1
  Read Car5 acc5/1 -> [a5], Display10/1
  Read Car5 dist/1 -> Sum4/2
  Read Car6 vel/1 -> [v6], Display12/1
  Read Car6 acc/1 -> [a6], Display13/1
  Read Car7 vel1/1 -> [v7], Display15/1
  Read Car7 acc1/1 -> [a7], Display16/1
  Read Car8 vel/1 -> [v8], Display18/1
  Read Car8 acc/1 -> [a8], Display19/1
  Read Car8 dist/1 -> Sum7/2
  Read Car9 vel/1 -> [v9], Display21/1
  Read Car9 acc/1 -> [a9], Display22/1
  Read Car10 vel/1 -> [v10], Display24/1
  Read Car10 acc/1 -> [a10], Display25/1
  Read Car10 dist/1 -> Sum9/2
  Read Car11 vel/1 -> [v11], Display27/1
  Read Car11 acc/1 -> [a11], Display28/1
  Read Car11 dist/1 -> Sum10/2
  Read Car12 vel/1 -> [v12], Display30/1
  Read Car12 acc/1 -> [a12], Display31/1
  Read Car12 dist/1 -> Sum11/2
  Read Car13 vel/1 -> [v13], Display33/1
  Read Car13 acc/1 -> [a13], Display34/1
  Read Car13 dist/1 -> Sum12/2
  Read Car14 vel/1 -> [v14], Display36/1
  Read Car14 acc/1 -> [a14], Display37/1
  Read Car14 dist/1 -> Sum13/2
  Read Car15 vel/1 -> [v15], Display39/1
  Read Car15 acc/1 -> [a15], Display40/1
  Read Car15 dist/1 -> Sum14/2
  Read Car16 vel/1 -> [v16], Display42/1
  Read Car16 acc/1 -> [a16], Display43/1
  Read Car16 dist/1 -> Sum15/2
  Read Car17 vel/1 -> [v17], Display45/1
  Read Car17 acc/1 -> [a17], Display46/1
  Read Car17 dist/1 -> Sum16/2
  Read Car18 vel/1 -> [v18], Display48/1
  Read Car18 acc/1 -> [a18], Display49/1
  Read Car18 dist/1 -> Sum17/2
  Read Car19 vel/1 -> [v19], Display51/1
  Read Car19 acc/1 -> [a19], Display52/1
  Read Car19 dist/1 -> Sum18/2
  Read Car20 vel/1 -> [v20], Display54/1
  Read Car20 acc/1 -> [a20], Display55/1
  Read Car20 dist/1 -> Sum19/2
  Mux/1 -> "S "/1
  Mux1/1 -> "V "/1
  [s2] -> Mux/2
  [s3] -> Mux/3
  [s8] -> Mux/8
  [s18] -> Mux/18
  [s6] -> Mux/6
  [s19] -> Mux/19
  [s13] -> Mux/13
  [s7] -> Mux/7
  [s4] -> Mux/4
  [s17] -> Mux/17
  [s12] -> Mux/12
  [s11] -> Mux/11
  [s20] -> Mux/20
  [s10] -> Mux/10
  [s16] -> Mux/16
  [s5] -> Mux/5
  [s14] -> Mux/14
  [s15] -> Mux/15
  [s9] -> Mux/9
  [v15] -> Mux1/15
  [v5] -> Mux1/5
  [v20] -> Mux1/20
  [v12] -> Mux1/12
  [v7] -> Mux1/7
  [v2] -> Mux1/2
  [v9] -> Mux1/9
  [v18] -> Mux1/18
  [v17] -> Mux1/17
  [v16] -> Mux1/16
  [v10] -> Mux1/10
  [v3] -> Mux1/3
  [v11] -> Mux1/11
  [v1] -> Mux1/1
  [v8] -> Mux1/8
  [v13] -> Mux1/13
  [v14] -> Mux1/14
  [v4] -> Mux1/4
  [v19] -> Mux1/19
  [v6] -> Mux1/6
  [a2] -> Mux2/2
  [a3] -> Mux2/3
  [a4] -> Mux2/4
  [a5] -> Mux2/5
  [a6] -> Mux2/6
  [a7] -> Mux2/7
  [a8] -> Mux2/8
  [a9] -> Mux2/9
  [a10] -> Mux2/10
  [a11] -> Mux2/11
  [a12] -> Mux2/12
  [a13] -> Mux2/13
  [a14] -> Mux2/14
  [a15] -> Mux2/15
  [a16] -> Mux2/16
  [a17] -> Mux2/17
  [a18] -> Mux2/18
  [a19] -> Mux2/19
  [a20] -> Mux2/20
  Mux2/1 -> "A "/1
  Read CM acceleration/1 -> [a1], vx1/1
  Read CM velocity/1 -> [v1], vx2/1
  [s1] -> Mux/1
  [a1] -> Mux2/1
  Constant/1 -> Sum/1
  "Read CM position "/1 -> Sum/2
  Sum/1 -> pos/1, [s1]
  Constant1/1 -> Sum1/1
  Sum1/1 -> Display1/1, [s2]
  Constant2/1 -> Sum2/1
  Sum2/1 -> Display3/1, [s3]
  Constant3/1 -> Sum3/1
  Sum3/1 -> Display8/1, [s4]
  Constant4/1 -> Sum4/1
  Sum4/1 -> Display11/1, [s5]
  Constant5/1 -> Sum5/1
  Sum5/1 -> Display14/1, [s6]
  Read Car6 dist/1 -> Sum5/2
  Constant6/1 -> Sum6/1
  Read Car7 dist1/1 -> Sum6/2
  Sum6/1 -> Display17/1, [s7]
  Constant7/1 -> Sum7/1
  Sum7/1 -> Display20/1, [s8]
  Constant8/1 -> Sum8/1
  Read Car9 dist/1 -> Sum8/2
  Sum8/1 -> Display23/1, [s9]
  Constant9/1 -> Sum9/1
  Sum9/1 -> Display26/1, [s10]
  Constant10/1 -> Sum10/1
  Sum10/1 -> Display29/1, [s11]
  Constant11/1 -> Sum11/1
  Sum11/1 -> Display32/1, [s12]
  Constant12/1 -> Sum12/1
  Sum12/1 -> Display35/1, [s13]
  Constant13/1 -> Sum13/1
  Sum13/1 -> Display38/1, [s14]
  Constant14/1 -> Sum14/1
  Sum14/1 -> Display41/1, [s15]
  Constant15/1 -> Sum15/1
  Sum15/1 -> Display44/1, [s16]
  Constant16/1 -> Sum16/1
  Sum16/1 -> Display47/1, [s17]
  Constant17/1 -> Sum17/1
  Sum17/1 -> Display50/1, [s18]
  Constant18/1 -> Sum18/1
  Sum18/1 -> Display53/1, [s19]
  Constant19/1 -> Sum19/1
  Sum19/1 -> Display56/1, [s20]

== system generic_wilmer_och_linnea_medvektorer2016b/CarMaker/IPG Vehicle/Brake/CreateBus Vhcl.Wheel.PT ==
  In : Inport
  BusCreator : BusCreator  Inputs=16
  Demux : Demux  Outputs=16
  Out : Outport
  wires:
  Demux/16 -> BusCreator/16  "Vhcl Wheel RR WhlBearing"
  Demux/15 -> BusCreator/15  "Vhcl Wheel RR Trq_T2W"
  Demux/14 -> BusCreator/14  "Vhcl Wheel RR Trq_BrakeReg_trg"
  Demux/13 -> BusCreator/13  "Vhcl Wheel RR Trq_Brake"
  Demux/12 -> BusCreator/12  "Vhcl Wheel RL WhlBearing"
  Demux/11 -> BusCreator/11  "Vhcl Wheel RL Trq_T2W"
  Demux/10 -> BusCreator/10  "Vhcl Wheel RL Trq_BrakeReg_trg"
  Demux/9 -> BusCreator/9  "Vhcl Wheel RL Trq_Brake"
  Demux/8 -> BusCreator/8  "Vhcl Wheel FR WhlBearing"
  Demux/7 -> BusCreator/7  "Vhcl Wheel FR Trq_T2W"
  Demux/6 -> BusCreator/6  "Vhcl Wheel FR Trq_BrakeReg_trg"
  Demux/5 -> BusCreator/5  "Vhcl Wheel FR Trq_Brake"
  Demux/4 -> BusCreator/4  "Vhcl Wheel FL WhlBearing"
  Demux/3 -> BusCreator/3  "Vhcl Wheel FL Trq_T2W"
  Demux/2 -> BusCreator/2  "Vhcl Wheel FL Trq_BrakeReg_trg"
  Demux/1 -> BusCreator/1  "Vhcl Wheel FL Trq_Brake"
  BusCreator/1 -> Out/1
  In/1 -> Demux/1

== system generic_wilmer_och_linnea_medvektorer2016b/CarMaker/IPG Vehicle/CarAndTrailer/CarAndTrailerUpd ==
  Sync_In : Inport
  Vhcl.Steering : Inport  Port=2
  Vhcl.Motion : Inport  Port=3
  Vhcl.PoI : Inport  Port=4
  Vhcl.Wheel.FL : Inport  Port=5
  Vhcl.Wheel.FR : Inport  Port=6
  Vhcl.Wheel.RL : Inport  Port=7
  Vhcl.Wheel.RR : Inport  Port=8
  Car.Hitch.FrcTrq : Inport  Port=9
  Vhcl.Fr1A : Inport  Port=10
  CarAndTrailerUpd : S-Function  FunctionName=CM_Sfun  Parameters='CarAndTrUpd'  SFunctionDeploymentMode=off  EnableBusSupport=off
  CreateBus Brake.IF.In : Subsystem
  Sync_Out : Outport
  Brake.IF.In : Outport  Port=2
  wires:
  Vhcl.Fr1A/1 -> CarAndTrailerUpd/10  "user vehicle only"
  Vhcl.Steering/1 -> CarAndTrailerUpd/2
  Vhcl.Motion/1 -> CarAndTrailerUpd/3
  Vhcl.PoI/1 -> CarAndTrailerUpd/4
  Vhcl.Wheel.FL/1 -> CarAndTrailerUpd/5
  Vhcl.Wheel.FR/1 -> CarAndTrailerUpd/6
  Car.Hitch.FrcTrq/1 -> CarAndTrailerUpd/9
  Vhcl.Wheel.RR/1 -> CarAndTrailerUpd/8
  Vhcl.Wheel.RL/1 -> CarAndTrailerUpd/7
  CarAndTrailerUpd/2 -> CreateBus Brake.IF.In/1(In)
  CreateBus Brake.IF.In/1(Out) -> Brake.IF.In/1
  CarAndTrailerUpd/1 -> Sync_Out/1
  Sync_In/1 -> CarAndTrailerUpd/1

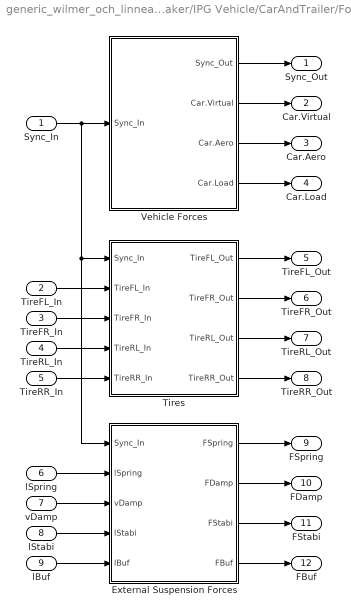
== system generic_wilmer_och_linnea_medvektorer2016b/CarMaker/IPG Vehicle/CarAndTrailer/Forces ==
  Sync_In : Inport
  TireFL_In : Inport  Port=2
  TireFR_In : Inport  Port=3
  TireRL_In : Inport  Port=4
  TireRR_In : Inport  Port=5
  lSpring : Inport  Port=6
  vDamp : Inport  Port=7
  lStabi : Inport  Port=8
  lBuf : Inport  Port=9
  External Suspension Forces : Subsystem
  Tires : Subsystem
  Vehicle Forces : Subsystem
  Sync_Out : Outport
  Car.Virtual : Outport  Port=2
  Car.Aero : Outport  Port=3
  Car.Load : Outport  Port=4
  TireFL_Out : Outport  Port=5
  TireFR_Out : Outport  Port=6
  TireRL_Out : Outport  Port=7
  TireRR_Out : Outport  Port=8
  FSpring : Outport  Port=9
  FDamp : Outport  Port=10
  FStabi : Outport  Port=11
  FBuf : Outport  Port=12
  wires:
  External Suspension Forces/4(FBuf) -> FBuf/1
  lBuf/1 -> External Suspension Forces/5(lBuf)
  Tires/4(TireRR_Out) -> TireRR_Out/1
  Tires/3(TireRL_Out) -> TireRL_Out/1
  Tires/2(TireFR_Out) -> TireFR_Out/1
  Tires/1(TireFL_Out) -> TireFL_Out/1
  TireRR_In/1 -> Tires/5(TireRR_In)
  TireRL_In/1 -> Tires/4(TireRL_In)
  TireFR_In/1 -> Tires/3(TireFR_In)
  Sync_In/1 -> External Suspension Forces/1(Sync_In), Tires/1(Sync_In), Vehicle Forces/1(Sync_In)
  Vehicle Forces/1(Sync_Out) -> Sync_Out/1
  TireFL_In/1 -> Tires/2(TireFL_In)
  Vehicle Forces/2(Car.Virtual) -> Car.Virtual/1
  Vehicle Forces/3(Car.Aero) -> Car.Aero/1
  Vehicle Forces/4(Car.Load) -> Car.Load/1
  lSpring/1 -> External Suspension Forces/2(lSpring)
  External Suspension Forces/2(FDamp) -> FDamp/1
  vDamp/1 -> External Suspension Forces/3(vDamp)
  lStabi/1 -> External Suspension Forces/4(lStabi)
  External Suspension Forces/3(FStabi) -> FStabi/1
  External Suspension Forces/1(FSpring) -> FSpring/1

== system generic_wilmer_och_linnea_medvektorer2016b/CarMaker/IPG Vehicle/CarAndTrailer/Kinematics ==
  Sync_In : Inport
  Steer.IF : Inport  Port=2
  Kinematics : S-Function  FunctionName=CM_Sfun  Parameters='Kinematics'  SFunctionDeploymentMode=off  EnableBusSupport=off
  Sync_Out : Outport
  TireFL_In : Outport  Port=2
  TireFR_In : Outport  Port=3
  TireRL_In : Outport  Port=4
  TireRR_In : Outport  Port=5
  lSpring : Outport  Port=6
  vDamp : Outport  Port=7
  lStabi : Outport  Port=8
  lBuf : Outport  Port=9
  wires:
  Kinematics/9 -> lBuf/1
  Kinematics/8 -> lStabi/1
  Kinematics/2 -> TireFL_In/1
  Kinematics/3 -> TireFR_In/1
  Kinematics/4 -> TireRL_In/1
  Kinematics/5 -> TireRR_In/1
  Kinematics/6 -> lSpring/1
  Kinematics/7 -> vDamp/1
  Sync_In/1 -> Kinematics/1
  Kinematics/1 -> Sync_Out/1
  Steer.IF/1 -> Kinematics/2

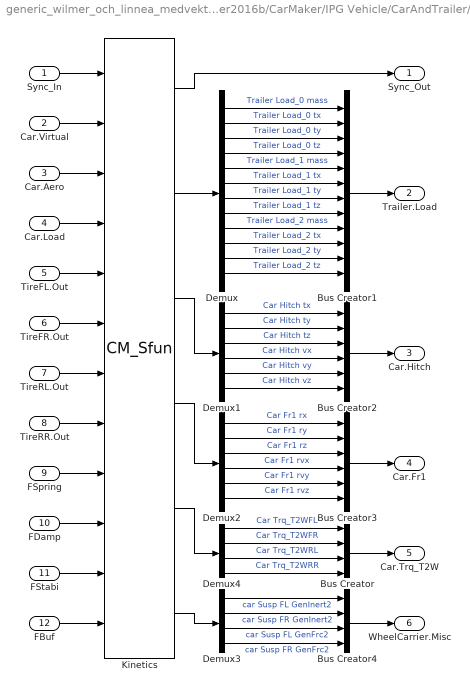
== system generic_wilmer_och_linnea_medvektorer2016b/CarMaker/IPG Vehicle/CarAndTrailer/Kinetics ==
  Sync_In : Inport
  Car.Virtual : Inport  Port=2
  Car.Aero : Inport  Port=3
  Car.Load : Inport  Port=4
  TireFL.Out : Inport  Port=5
  TireFR.Out : Inport  Port=6
  TireRL.Out : Inport  Port=7
  TireRR.Out : Inport  Port=8
  FSpring : Inport  Port=9
  FDamp : Inport  Port=10
  FStabi : Inport  Port=11
  FBuf : Inport  Port=12
  Bus Creator : BusCreator  Inputs=4
  Bus Creator1 : BusCreator  Inputs=12
  Bus Creator2 : BusCreator  Inputs=6
  Bus Creator3 : BusCreator  Inputs=6
  Bus Creator4 : BusCreator  Inputs=4
  Demux : Demux  Outputs=12
  Demux1 : Demux  Outputs=6
  Demux2 : Demux  Outputs=6
  Demux3 : Demux
  Demux4 : Demux
  Kinetics : S-Function  FunctionName=CM_Sfun  Parameters='Kinetics'  SFunctionDeploymentMode=off  EnableBusSupport=off
  Sync_Out : Outport
  Trailer.Load : Outport  Port=2
  Car.Hitch : Outport  Port=3
  Car.Fr1 : Outport  Port=4
  Car.Trq_T2W : Outport  Port=5
  WheelCarrier.Misc : Outport  Port=6
  wires:
  FBuf/1 -> Kinetics/12
  Sync_In/1 -> Kinetics/1
  Kinetics/1 -> Sync_Out/1
  Car.Aero/1 -> Kinetics/3
  Car.Virtual/1 -> Kinetics/2
  Bus Creator1/1 -> Trailer.Load/1
  Demux/1 -> Bus Creator1/1  "Trailer Load_0 mass"
  Demux/2 -> Bus Creator1/2  "Trailer Load_0 tx"
  Demux/3 -> Bus Creator1/3  "Trailer Load_0 ty"
  Demux/4 -> Bus Creator1/4  "Trailer Load_0 tz"
  Kinetics/2 -> Demux/1
  Demux/5 -> Bus Creator1/5  "Trailer Load_1 mass"
  Demux/6 -> Bus Creator1/6  "Trailer Load_1 tx"
  Demux/7 -> Bus Creator1/7  "Trailer Load_1 ty"
  Demux/8 -> Bus Creator1/8  "Trailer Load_1 tz"
  Demux/9 -> Bus Creator1/9  "Trailer Load_2 mass"
  Demux/10 -> Bus Creator1/10  "Trailer Load_2 tx"
  Demux/11 -> Bus Creator1/11  "Trailer Load_2 ty"
  Demux/12 -> Bus Creator1/12  "Trailer Load_2 tz"
  Demux1/1 -> Bus Creator2/1  "Car Hitch tx"
  Demux1/2 -> Bus Creator2/2  "Car Hitch ty"
  Demux1/3 -> Bus Creator2/3  "Car Hitch tz"
  Demux1/4 -> Bus Creator2/4  "Car Hitch vx"
  Demux1/5 -> Bus Creator2/5  "Car Hitch vy"
  Demux1/6 -> Bus Creator2/6  "Car Hitch vz"
  Kinetics/3 -> Demux1/1
  Bus Creator2/1 -> Car.Hitch/1
  Demux2/1 -> Bus Creator3/1  "Car Fr1 rx"
  Demux2/2 -> Bus Creator3/2  "Car Fr1 ry"
  Demux2/3 -> Bus Creator3/3  "Car Fr1 rz"
  Demux2/4 -> Bus Creator3/4  "Car Fr1 rvx"
  Demux2/5 -> Bus Creator3/5  "Car Fr1 rvy"
  Demux2/6 -> Bus Creator3/6  "Car Fr1 rvz"
  Bus Creator3/1 -> Car.Fr1/1
  Kinetics/4 -> Demux2/1
  Car.Load/1 -> Kinetics/4
  Demux3/1 -> Bus Creator4/1  "car Susp FL GenInert2"
  Demux3/2 -> Bus Creator4/2  "car Susp FR GenInert2"
  Demux3/3 -> Bus Creator4/3  "car Susp FL GenFrc2"
  Demux3/4 -> Bus Creator4/4  "car Susp FR GenFrc2"
  Bus Creator4/1 -> WheelCarrier.Misc/1
  Bus Creator/1 -> Car.Trq_T2W/1
  Demux4/4 -> Bus Creator/4  "Car Trq_T2WRR"
  Demux4/3 -> Bus Creator/3  "Car Trq_T2WRL"
  Demux4/2 -> Bus Creator/2  "Car Trq_T2WFR"
  Demux4/1 -> Bus Creator/1  "Car Trq_T2WFL"
  TireFL.Out/1 -> Kinetics/5
  TireFR.Out/1 -> Kinetics/6
  TireRL.Out/1 -> Kinetics/7
  TireRR.Out/1 -> Kinetics/8
  FSpring/1 -> Kinetics/9
  FDamp/1 -> Kinetics/10
  FStabi/1 -> Kinetics/11
  Kinetics/6 -> Demux3/1
  Kinetics/5 -> Demux4/1

== system generic_wilmer_och_linnea_medvektorer2016b/CarMaker/IPG Vehicle/CarAndTrailer/Steering ==
  note: When replacing the entire steering system,
      | be sure to add '-disablesteering' to the command line arguments
      | in the CarMaker Model Configuration block.
  Sync_In : Inport
  VhclCtrl.Steering : Inport  Port=2
  Bus Creator1 : BusCreator  Inputs=16
  Bus Creator2 : BusCreator  Inputs=4
  Demux : Demux  Outputs=20
  Steering : S-Function  FunctionName=CM_Sfun  Parameters='Steering'  SFunctionDeploymentMode=off  EnableBusSupport=off
  Terminator : Terminator
  Sync_Out : Outport
  Steer.IF : Outport  Port=2
  wires:
  Bus Creator1/1 -> Steer.IF/1
  Steering/2 -> Demux/1
  Demux/8 -> Bus Creator1/8  "Steering IF AssistTrqPin"
  Demux/7 -> Bus Creator1/7  "Steering IF AssistTrqCol"
  Demux/6 -> Bus Creator1/6  "Steering IF AssistFrc"
  Demux/20 -> Bus Creator2/4  "Steering IF R Inert"
  Demux/17 -> Bus Creator2/1  "Steering IF L Frc"
  Demux/18 -> Bus Creator2/2  "Steering IF L Inert"
  Demux/19 -> Bus Creator2/3  "Steering IF R Frc"
  Bus Creator2/1 -> Terminator/1  "Steer IF (in)"
  Demux/16 -> Bus Creator1/16  "Steering IF R iSteer2q"
  Demux/9 -> Bus Creator1/9  "Steering IF L q"
  Demux/10 -> Bus Creator1/10  "Steering IF L qp"
  Demux/11 -> Bus Creator1/11  "Steering IF L qpp"
  Demux/12 -> Bus Creator1/12  "Steering IF L iSteer2q"
  Demux/13 -> Bus Creator1/13  "Steering IF R q"
  Demux/14 -> Bus Creator1/14  "Steering IF R qp"
  Demux/15 -> Bus Creator1/15  "Steering IF R qpp"
  VhclCtrl.Steering/1 -> Steering/2
  Steering/1 -> Sync_Out/1
  Sync_In/1 -> Steering/1
  Demux/1 -> Bus Creator1/1  "Steering IF Ang"
  Demux/2 -> Bus Creator1/2  "Steering IF AngVel"
  Demux/3 -> Bus Creator1/3  "Steering IF AngAcc"
  Demux/4 -> Bus Creator1/4  "Steering IF Trq"
  Demux/5 -> Bus Creator1/5  "Steering IF TrqStatic"

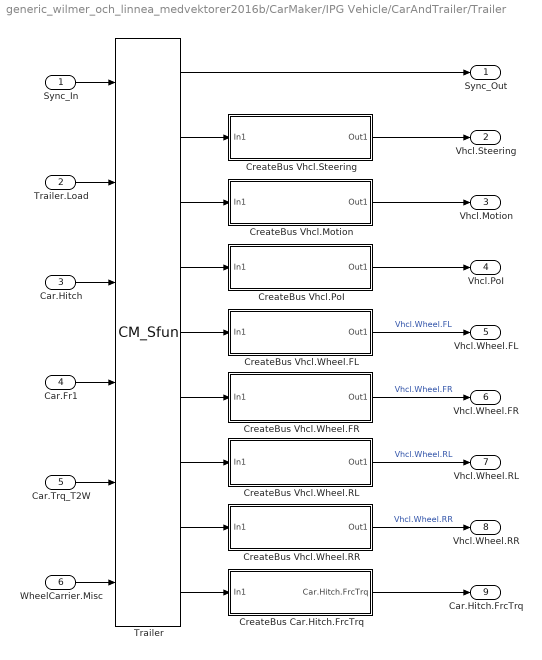
== system generic_wilmer_och_linnea_medvektorer2016b/CarMaker/IPG Vehicle/CarAndTrailer/Trailer ==
  Sync_In : Inport
  Trailer.Load : Inport  Port=2
  Car.Hitch : Inport  Port=3
  Car.Fr1 : Inport  Port=4
  Car.Trq_T2W : Inport  Port=5
  WheelCarrier.Misc : Inport  Port=6
  CreateBus Car.Hitch.FrcTrq : Subsystem
  CreateBus Vhcl.Motion : Subsystem
  CreateBus Vhcl.PoI : Subsystem
  CreateBus Vhcl.Steering : Subsystem
  CreateBus Vhcl.Wheel.FL : Subsystem
  CreateBus Vhcl.Wheel.FR : Subsystem
  CreateBus Vhcl.Wheel.RL : Subsystem
  CreateBus Vhcl.Wheel.RR : Subsystem
  Trailer : S-Function  FunctionName=CM_Sfun  Parameters='Trailer'  SFunctionDeploymentMode=off  EnableBusSupport=off
  Sync_Out : Outport
  Vhcl.Steering : Outport  Port=2
  Vhcl.Motion : Outport  Port=3
  Vhcl.PoI : Outport  Port=4
  Vhcl.Wheel.FL : Outport  Port=5
  Vhcl.Wheel.FR : Outport  Port=6
  Vhcl.Wheel.RL : Outport  Port=7
  Vhcl.Wheel.RR : Outport  Port=8
  Car.Hitch.FrcTrq : Outport  Port=9
  wires:
  Trailer/2 -> CreateBus Vhcl.Steering/1(In1)
  CreateBus Vhcl.Steering/1(Out1) -> Vhcl.Steering/1
  Trailer/3 -> CreateBus Vhcl.Motion/1(In1)
  Trailer/4 -> CreateBus Vhcl.PoI/1(In1)
  Trailer/5 -> CreateBus Vhcl.Wheel.FL/1(In1)
  Trailer/6 -> CreateBus Vhcl.Wheel.FR/1(In1)
  Trailer/7 -> CreateBus Vhcl.Wheel.RL/1(In1)
  Trailer/9 -> CreateBus Car.Hitch.FrcTrq/1(In1)
  Trailer/8 -> CreateBus Vhcl.Wheel.RR/1(In1)
  CreateBus Vhcl.Wheel.RR/1(Out1) -> Vhcl.Wheel.RR/1  "Vhcl.Wheel.RR"
  CreateBus Vhcl.Wheel.RL/1(Out1) -> Vhcl.Wheel.RL/1  "Vhcl.Wheel.RL"
  CreateBus Vhcl.Wheel.FR/1(Out1) -> Vhcl.Wheel.FR/1  "Vhcl.Wheel.FR"
  CreateBus Vhcl.Wheel.FL/1(Out1) -> Vhcl.Wheel.FL/1  "Vhcl.Wheel.FL"
  CreateBus Vhcl.PoI/1(Out1) -> Vhcl.PoI/1
  CreateBus Vhcl.Motion/1(Out1) -> Vhcl.Motion/1
  Car.Trq_T2W/1 -> Trailer/5
  WheelCarrier.Misc/1 -> Trailer/6
  CreateBus Car.Hitch.FrcTrq/1(Car.Hitch.FrcTrq) -> Car.Hitch.FrcTrq/1
  Car.Fr1/1 -> Trailer/4
  Car.Hitch/1 -> Trailer/3
  Trailer.Load/1 -> Trailer/2
  Trailer/1 -> Sync_Out/1
  Sync_In/1 -> Trailer/1

== system generic_wilmer_och_linnea_medvektorer2016b/CarMaker/VehicleControl/AccelCtrl1/PI-Controller ==
  delta_ax : Inport
  DM_Gas : Inport  Port=2
  AxCtrl On : Inport  Port=3
  Add : Sum  SaturateOnIntegerOverflow=on  OutDataTypeStr=Inherit: Same as first input
  I -gain : Display
  I Gain : Constant  Value=0.001
  Integrator : Subsystem
  P -gain : Display
  P -gain1 : Display
  P -gain2 : Display
  P Gain : Constant  Value=0.01
  Read init i_gain from Inf : CarMaker4SL/Read CM Parameter  xfile=Vehicle  xkey=AccelCtrl.i_gain  xnout=1  xdefaults=0.001  xmuxed=off
  Read init p_gain from Inf : CarMaker4SL/Read CM Parameter  xfile=Vehicle  xkey=AccelCtrl.p_gain  xnout=1  xdefaults=0.001  xmuxed=off
  Saturation : Saturate  UpperLimit=1  LowerLimit=-1
  i_gain : Product  SaturateOnIntegerOverflow=on  OutDataTypeStr=Inherit: Same as first input
  p_gain : Product  SaturateOnIntegerOverflow=on  OutDataTypeStr=Inherit: Same as first input
  Gas or Brake : Outport
  wires:
  I Gain/1 -> I -gain/1, i_gain/2
  P Gain/1 -> P -gain/1, p_gain/1
  Integrator/1("I-part tot ") -> Add/2
  DM_Gas/1 -> Integrator/3(Init I-part)
  AxCtrl On/1 -> Integrator/2(AxCtrl On)
  i_gain/1 -> Integrator/1(I-Part)
  delta_ax/1 -> i_gain/1, p_gain/2
  p_gain/1 -> Add/1
  Add/1 -> Saturation/1
  Saturation/1 -> Gas or Brake/1
  Read init p_gain from Inf/1 -> P -gain1/1
  Read init i_gain from Inf/1 -> P -gain2/1
